simulink library "cac"  (Simulink 8.1)
settings: Solver=ode1  StartTime=0.0  StopTime=Inf  FixedStep=0.001  RelTol=1e-3
PostLoadFcn:
  | , if any(exist('dsrtsu_mdlpostloadfcn', 'file') == [2, 3, 6]), try dsrtsu_mdlpostloadfcn('Execute', bdroot); catch fprintf('Error in PostLoadFcn (dsrtsu_mdlpostloadfcn) for model "%s":\n %s\n', bdroot, lasterr); end, end,
undefined symbols (not defined in the file or in its folder): FALSE, ZERO_FLOAT
libraries: cbc x1, hrc x1, slc x1, ctc x1
settings Model: DSRTSU_INTERNAL_RTI_VER=450  DSRTSU_INTERNAL_RTI_TYPE=rti1401  RTICANMMDATA=struct('GeneralSetupData',struct('modelroot','D:\ELN150201_TAIWAN\trunk\AdasDragon\software\sw_development\arch\app\acc','generalsettings',struct('filesettings',struct('destfolder',struct('Name','RTICANMM_FILES','Check',1),'buildfolder',struct('Name','.','Check',1),'AbsDestfolder',struct('Name','D:\ELN150201_TAIWAN\trunk\AdasDragon\software\sw_development\arch\app\acc\RTICANMM_FILES'),'AbsBuildfolder',struct('Name','D:\ELN150201_TAIWAN\trunk\AdasDragon\software\sw_development\arch\app\acc'))),'options',struct('addpaths',1,'rmpaths',1,'addtrcexclusion',logical(1),'cannavigator',struct('checkmonitoring',0),'show_usrtrc',0,'use_usrtrc',0),'advanced',struct('options',[1 1 1 1 1 1 1 1 1 1 1 1 1 1 1 1 1 1 1 1 1 1 1 1 1 1 1 1 1 1 1 1 1 1 1 1 1 1 1 1 1 1 1 1 1 1 1 1 1 1 1 1 1 1 1 1 1 1 1 1 1 1 1 1 1 1 1 1 1 1 1 1 1 1 1 1 1 1 1 1 1 1 1 1 1 1 1 1 1 1 1 1 1 1 1 1 1 1 1 1]),'MPSetup',{{}},'modelname','cac','block','cac'))  DSRTSU_INTERNAL_RTIFPGA=40  Creator=AT015411  LastModifiedBy=AT015555

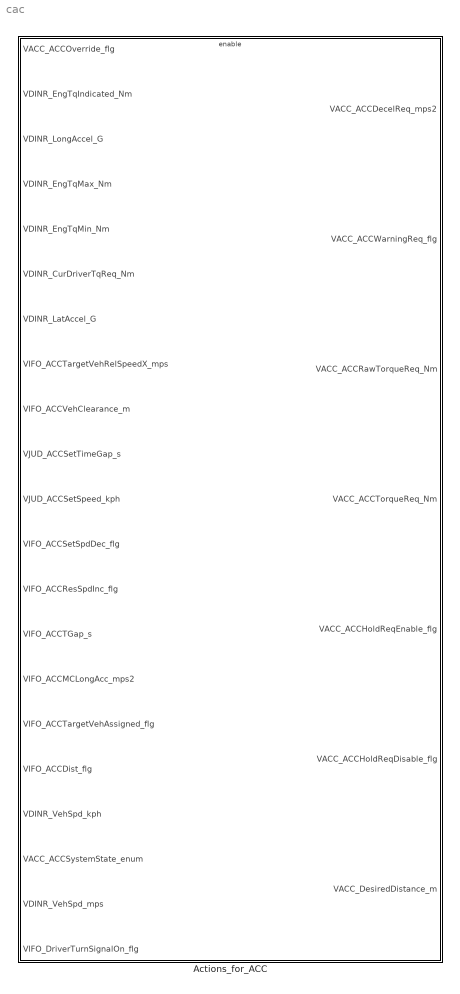
== system cac ==
  Actions_for_ACC : Subsystem

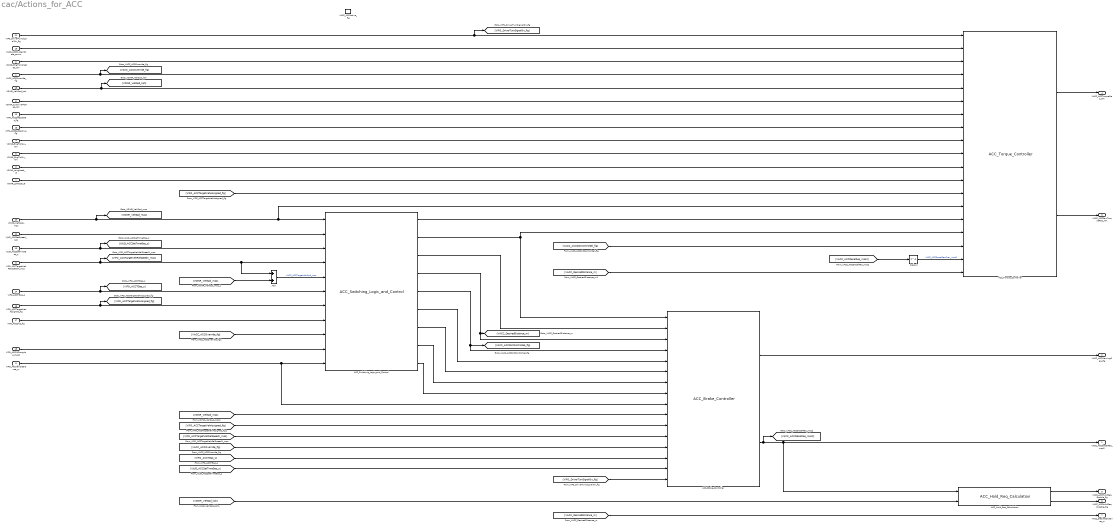
== system cac/Actions_for_ACC ==
  VACC_ACCOverride_flg : Inport
  VDINR_EngTqIndicated_Nm : Inport  Port=2
  VDINR_LongAccel_G : Inport  Port=3
  VDINR_EngTqMax_Nm : Inport  Port=4
  VDINR_EngTqMin_Nm : Inport  Port=5
  VDINR_CurDriverTqReq_Nm : Inport  Port=6
  VDINR_LatAccel_G : Inport  Port=7
  VIFO_ACCTargetVehRelSpeedX_mps : Inport  Port=8
  VIFO_ACCVehClearance_m : Inport  Port=9
  VJUD_ACCSetTimeGap_s : Inport  Port=10
  VJUD_ACCSetSpeed_kph : Inport  Port=11
  VIFO_ACCSetSpdDec_flg : Inport  Port=12
  VIFO_ACCResSpdInc_flg : Inport  Port=13
  VIFO_ACCTGap_s : Inport  Port=14
  VIFO_ACCMCLongAcc_mps2 : Inport  Port=15
  VIFO_ACCTargetVehAssigned_flg : Inport  Port=16
  VIFO_ACCDist_flg : Inport  Port=17
  VDINR_VehSpd_kph : Inport  Port=18
  VACC_ACCSystemState_enum : Inport  Port=19
  VDINR_VehSpd_mps : Inport  Port=20
  VIFO_DriverTurnSignalOn_flg : Inport  Port=21
  VACC_ACCActive_flg : EnablePort  StatesWhenEnabling=reset
      settings: AttributesFormatString=State=%<StatesWhenEnabling>
  ACC_Brake_Controller : cbc/ACC_Brake_Controller
  ACC_Hold_Req_Calculation : hrc/ACC_Hold_Req_Calculation
  ACC_Switching_Logic_and_Control : slc/ACC_Switching_Logic_and_Control
  ACC_Torque_Controller : ctc/ACC_Torque_Controller
  Add : Sum
  Delay2 : Delay  DelayLength=1  InitialCondition=0
  VACC_ACCDecelReq_mps2 : Outport  OutputWhenDisabled=reset  InitialOutput=ZERO_FLOAT
  VACC_ACCWarningReq_flg : Outport  Port=2  OutputWhenDisabled=reset  InitialOutput=FALSE
  VACC_ACCRawTorqueReq_Nm : Outport  Port=3  OutputWhenDisabled=reset  InitialOutput=ZERO_FLOAT
  VACC_ACCTorqueReq_Nm : Outport  Port=4  OutputWhenDisabled=reset  InitialOutput=ZERO_FLOAT
  VACC_ACCHoldReqEnable_flg : Outport  Port=5  OutputWhenDisabled=reset  InitialOutput=FALSE
  VACC_ACCHoldReqDisable_flg : Outport  Port=6  OutputWhenDisabled=reset  InitialOutput=FALSE
  VACC_DesiredDistance_m : Outport  Port=7  OutputWhenDisabled=reset  InitialOutput=FALSE
  wires:
  VDINR_EngTqIndicated_Nm/1 -> ACC_Torque_Controller/3
  VIFO_ACCDist_flg/1 -> ACC_Switching_Logic_and_Control/8
  VIFO_ACCVehClearance_m/1 -> ACC_Brake_Controller/9, ACC_Switching_Logic_and_Control/11
  [VDINR_VehSpd_mps] -> Add/2
  VDINR_VehSpd_mps/1 -> [VDINR_VehSpd_mps], ACC_Torque_Controller/14, ACC_Switching_Logic_and_Control/1
  VIFO_ACCTargetVehAssigned_flg/1 -> ACC_Switching_Logic_and_Control/7, [VIFO_ACCTargetVehAssigned_flg]
  Add/1 -> ACC_Switching_Logic_and_Control/5  "VACC_ACCTargetVehSpd_mps"
  VIFO_ACCTargetVehRelSpeedX_mps/1 -> [VIFO_ACCTargetVehRelSpeedX_mps], Add/1, ACC_Switching_Logic_and_Control/4
  VJUD_ACCSetSpeed_kph/1 -> ACC_Switching_Logic_and_Control/2
  ACC_Hold_Req_Calculation/1 -> VACC_ACCHoldReqEnable_flg/1
  VDINR_LatAccel_G/1 -> ACC_Torque_Controller/12
  VACC_ACCOverride_flg/1 -> [VACC_ACCOverride_flg], ACC_Torque_Controller/4
  VDINR_LongAccel_G/1 -> ACC_Torque_Controller/11
  [VACC_ACCOverride_flg] -> ACC_Brake_Controller/13
  ACC_Torque_Controller/1 -> VACC_ACCTorqueReq_Nm/1
  VDINR_EngTqMin_Nm/1 -> ACC_Torque_Controller/10
  VDINR_EngTqMax_Nm/1 -> ACC_Torque_Controller/9
  [VDINR_VehSpd_mps] -> ACC_Brake_Controller/10
  [VIFO_ACCTargetVehRelSpeedX_mps] -> ACC_Brake_Controller/12
  ACC_Switching_Logic_and_Control/4 -> ACC_Brake_Controller/3, [VACC_DesiredDistance_m]
  ACC_Switching_Logic_and_Control/3 -> ACC_Brake_Controller/2
  ACC_Switching_Logic_and_Control/1 -> ACC_Torque_Controller/15
  VDINR_CurDriverTqReq_Nm/1 -> ACC_Torque_Controller/6
  VDINR_VehSpd_kph/1 -> [VDINR_VehSpd_kph], ACC_Torque_Controller/5
  VIFO_ACCSetSpdDec_flg/1 -> ACC_Torque_Controller/7
  VIFO_ACCResSpdInc_flg/1 -> ACC_Torque_Controller/8
  ACC_Torque_Controller/2 -> VACC_ACCRawTorqueReq_Nm/1
  ACC_Switching_Logic_and_Control/2 -> ACC_Brake_Controller/1, ACC_Torque_Controller/16
  [VACC_ACCOverride_flg] -> ACC_Switching_Logic_and_Control/9
  ACC_Hold_Req_Calculation/2 -> VACC_ACCHoldReqDisable_flg/1
  ACC_Brake_Controller/1 -> VACC_ACCWarningReq_flg/1
  ACC_Brake_Controller/2 -> VACC_ACCDecelReq_mps2/1, ACC_Hold_Req_Calculation/1, [VACC_ACCDecelReq_mps2]
  [VDINR_VehSpd_kph] -> ACC_Hold_Req_Calculation/2
  [VACC_DesiredDistance_m] -> VACC_DesiredDistance_m/1
  ACC_Switching_Logic_and_Control/5 -> ACC_Brake_Controller/4, [VACC_ACCDistControlSel_flg]
  [VACC_ACCDistControlSel_flg] -> ACC_Torque_Controller/17
  [VACC_ACCDecelReq_mps2] -> Delay2/1
  Delay2/1 -> ACC_Torque_Controller/18  "VACC_ACCDecelReqPrev_mps2"
  VIFO_ACCMCLongAcc_mps2/1 -> ACC_Switching_Logic_and_Control/10
  VACC_ACCSystemState_enum/1 -> ACC_Torque_Controller/2
  [VIFO_ACCTargetVehAssigned_flg] -> ACC_Torque_Controller/13
  [VIFO_ACCTargetVehAssigned_flg] -> ACC_Brake_Controller/11
  VIFO_ACCTGap_s/1 -> ACC_Switching_Logic_and_Control/6, [VIFO_ACCTGap_s]
  ACC_Switching_Logic_and_Control/6 -> ACC_Brake_Controller/5
  [VACC_DesiredDistance_m] -> ACC_Torque_Controller/19
  ACC_Switching_Logic_and_Control/7 -> ACC_Brake_Controller/6
  ACC_Switching_Logic_and_Control/8 -> ACC_Brake_Controller/7
  [VIFO_ACCTGap_s] -> ACC_Brake_Controller/14
  VJUD_ACCSetTimeGap_s/1 -> [VJUD_ACCSetTimeGap_s], ACC_Switching_Logic_and_Control/3
  [VJUD_ACCSetTimeGap_s] -> ACC_Brake_Controller/15
  VIFO_DriverTurnSignalOn_flg/1 -> [VIFO_DriverTurnSignalOn_flg], ACC_Torque_Controller/1
  [VIFO_DriverTurnSignalOn_flg] -> ACC_Brake_Controller/16
  ACC_Switching_Logic_and_Control/9 -> ACC_Brake_Controller/8
